simulink model "motor_dc_pid"  (R2018a)
settings: Solver=VariableStepAuto  StartTime=0.0  StopTime=10.0  RelTol=1e-3
values from neighbouring files (symbols this model uses):
  If = 1    [script_motor_cc.m]
  J = 0.001    [script_motor_cc.m]
  K1 = (M*If*In)/(2*pi*n/60)    (= 0.0222906604013)    [script_motor_cc.m]
  La = 0.0025    [script_motor_cc.m]
  M = (Vn - Ra*In)/(2*pi*n/60)/If    (= 0.350140874802)    [script_motor_cc.m]
  Ra = 0.5    [script_motor_cc.m]
  Vn = 120    [script_motor_cc.m]
  Vpwm = 565    [script_motor_cc.m]
libraries: powerlib x8, simulink x2, powerlib_meascontrol x1
settings Model: PauseTimes=1.5  Creator=Gustavo  LastModifiedBy=Gustavo

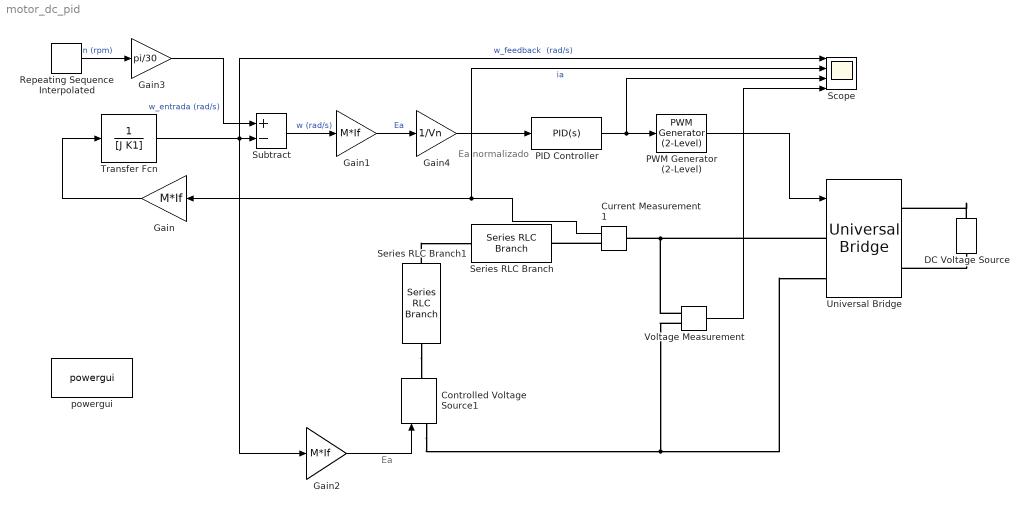
== system motor_dc_pid ==
  note: Ea normalizado
  note: Ea
  Controlled Voltage Source1 : powerlib/Electrical Sources/Controlled Voltage Source  Initialize=on  Source_Type=DC  Amplitude=Vn  Phase=0  Frequency=0  Measurements=None
  Current Measurement1 : powerlib/Measurements/Current Measurement  PhasorSimulation=off  OutputType=Complex  PSBequivalent=0
  DC Voltage Source : powerlib/Electrical Sources/DC Voltage Source  Amplitude=Vpwm  Measurements=None
  Gain : Gain  Gain=M*If
  Gain1 : Gain  Gain=M*If
  Gain2 : Gain  Gain=M*If
  Gain3 : Gain  Gain=pi/30
  Gain4 : Gain  Gain=1/Vn  OutDataTypeStr=double
  PID Controller : simulink/Continuous/PID Controller  Controller=PID  TimeDomain=Continuous-time  SampleTime=-1  IntegratorMethod=Forward Euler  FilterMethod=Forward Euler  Form=Parallel  UseFilter=on  ControllerParametersSource=internal  P=1  I=0  D=0  N=1  InitialConditionSource=internal  InitialConditionForIntegrator=0  InitialConditionForFilter=0  ExternalReset=none  LimitOutput=off  UpperSaturationLimit=0.20  LowerSaturationLimit=-0.20  LinearizeAsGain=on  AntiWindupMode=clamping  Kb=1  TrackingMode=off  Kt=1  PParamMin=[]  PParamMax=[]  IParamMin=[]  IParamMax=[]  DParamMin=[]  DParamMax=[]  NParamMin=[]  NParamMax=[]  KbParamMin=[]  KbParamMax=[]  KtParamMin=[]  KtParamMax=[]  POutMin=[]  POutMax=[]  IOutMin=[]  IOutMax=[]  DOutMin=[]  DOutMax=[]  NOutMin=[]  NOutMax=[]  KbOutMin=[]  KbOutMax=[]  KtOutMin=[]  KtOutMax=[]  IntegratorOutMin=[]  IntegratorOutMax=[]  FilterOutMin=[]  FilterOutMax=[]  SumOutMin=[]  SumOutMax=[]  SumI1OutMin=[]  SumI1OutMax=[]  SumI2OutMin=[]  SumI2OutMax=[]  SumI3OutMin=[]  SumI3OutMax=[]  SumDOutMin=[]  SumDOutMax=[]  SaturationOutMin=[]  SaturationOutMax=[]  IntegratorContinuousStateAttributes=''  IntegratorStateMustResolveToSignalObject=off  IntegratorRTWStateStorageClass=Auto  FilterContinuousStateAttributes=''  FilterStateMustResolveToSignalObject=off  FilterRTWStateStorageClass=Auto  DifferentiatorICPrevScaledInput=0  DifferentiatorOutMin=[]  DifferentiatorOutMax=[]  FilterDiffOutCoefMin=[]  FilterDiffOutCoefMax=[]  SumDenOutMin=[]  SumDenOutMax=[]  SumNumOutMin=[]  SumNumOutMax=[]  ReciprocalOutMin=[]  ReciprocalOutMax=[]  DivideOutMin=[]  DivideOutMax=[]  TunerSelectOption=Transfer Function Based (PID Tuner App)
  PWM Generator (2-Level) : powerlib_meascontrol/Pulse & Signal Generators/PWM Generator (2-Level)  ModulatorType=Single-phase full-bridge (4 pulses)  ModulatorMode=Unsynchronized  Fc=27*60  Pc=90  nF=27  MinMax="[ -1  1 ]"  SamplingTechnique=Natural  ModulatingSignals=off  m=0.8  Freq=60  Phase=0  Ts=0  ShowCarrierOutport=off
      settings: SourceProductName=Simscape Power Systems
  Repeating Sequence Interpolated : simulink/Sources/Repeating Sequence Interpolated  OutValues=w_desejado  TimeValues=t  LookUpMeth=Interpolation-Use End Values  tsamp=0.0001  OutMin=[]  OutMax=[]  OutDataTypeStr=double  OutputDataTypeScalingMode=double  OutDataType=fixdt(0,8)  OutScaling=2^-10
  Scope : Scope  NumInputPorts=4
  Series RLC Branch : powerlib/Elements/Series RLC Branch  LConnTagsString=__new0  RConnTagsString=__new0  BranchType=R  Resistance=Ra  Inductance=1e-3  SetiL0=off  InitialCurrent=0  Capacitance=1e-6  Setx0=off  InitialVoltage=0  Measurements=None
  Series RLC Branch1 : powerlib/Elements/Series RLC Branch  LConnTagsString=__new0  RConnTagsString=__new0  BranchType=L  Resistance=1  Inductance=La  SetiL0=on  InitialCurrent=20  Capacitance=1e-6  Setx0=off  InitialVoltage=0  Measurements=None
  Subtract : Sum  Inputs=+-
  Transfer Fcn : TransferFcn  Denominator=[J K1]
  Universal Bridge : powerlib/Power Electronics/Universal Bridge  Arms=2  SnubberResistance=1e5  SnubberCapacitance=inf  Device=MOSFET / Diodes  Ron=1e-3  Lon=0  ForwardVoltages="[  0  0  ]"  ForwardVoltage=0  GTOparameters=[ 10e-6 , 20e-6 ]  IGBTparameters=[ 1e-6 , 2e-6 ]  Measurements=None  Measurements_2=None  converterType=Rectifier
  Voltage Measurement : powerlib/Measurements/Voltage Measurement  PhasorSimulation=off  OutputType=Complex  PSBequivalent=0
  powergui : powerlib/powergui  Priority=1  SimulationMode=Continuous  SampleTime=50e-6  frequency=60  Iterations=50  frequencyindice=0  Pbase=100e6  ErrMax=1e-4  UnitsV=kV  UnitsW=MW  buscounter=0  FunctionMessages=off  echomessages=off  EnableUseOfTLC=off  CurrentSourceSwitches=off  DisableSnubberDevices=off  DisableRonSwitches=off  DisableVfSwitches=off  DisplayEquations=off  SolverType=Tustin/Backward Euler (TBE)  Interpol=off  ExternalGateDelay=off  methode=off  Ts=100  x0status=blocks  SPID=on  SwTol=0  HookPort=off  RestoreLinks=warning  ResistiveCurrentMeasurement=off  Frange=[0:2:500]  Ylog=off  Xlog=on  ShowGrid=off  save=off  variable=ZData  structure=0  ZoomFFT=off  StartTime=0.0  cycles=1  DisplayStyle=1  fundamental=60  FreqAxis=off  MaxFrequency=1000  frequencyindicesteady=1  RmsSteady=1  display=off
  wires:
  Gain/1 -> Transfer Fcn/1
  Subtract/1 -> Gain1/1  "w (rad/s)"
  Repeating Sequence Interpolated/1 -> Gain3/1  "n (rpm)"
  Gain1/1 -> Gain4/1  "Ea"
  Gain2/1 -> Controlled Voltage Source1/1
  Current Measurement1/1 -> Scope/2, Gain/1  "ia"
  PWM Generator (2-Level)/1 -> Universal Bridge/1
  Gain3/1 -> Subtract/1  "w_entrada (rad/s)"
  Transfer Fcn/1 -> Scope/1, Gain2/1, Subtract/2  "w_feedback  (rad/s)"
  Voltage Measurement/1 -> Scope/4
  Gain4/1 -> PID Controller/1
  PID Controller/1 -> Scope/3, PWM Generator (2-Level)/1
  connections:
  Current Measurement1/RConn1 -- Series RLC Branch/RConn1
  Voltage Measurement/LConn1 -- Current Measurement1/LConn1 -- Universal Bridge/LConn1
  Series RLC Branch1/RConn1 -- Controlled Voltage Source1/RConn1
  Series RLC Branch1/LConn1 -- Series RLC Branch/LConn1
  Controlled Voltage Source1/LConn1 -- Voltage Measurement/LConn2 -- Universal Bridge/LConn2
  DC Voltage Source/RConn1 -- Universal Bridge/RConn1
  DC Voltage Source/LConn1 -- Universal Bridge/RConn2
